simulink model "Demo_DSRC_BSM_Message_cs"  (Simulink 7.6)
settings: Solver=ode5  SolverMode=SingleTasking  StartTime=0.0  StopTime=10  FixedStep=1/20  RelTol=1e-3
model workspace (MAT data in the model file):
  mbox_table.block_array(1).src = 'built-in/Subsystem'
  mbox_table.block_array(1).dest = 'Demo_DSRC_BSM_Message_cs/BMW_Z3_1'
  mbox_table.block_array(1).mode = 0
  mbox_table.block_array(2).src = 'simulink/Sinks/Out1'
  mbox_table.block_array(2).dest = 'Demo_DSRC_BSM_Message_cs/BMW_Z3_1/STATE_BMW_Z3_1'
  mbox_table.block_array(2).mode = 0
  mbox_table.block_array(3).src = 'PreScanSimulinkLibrary/State'
  mbox_table.block_array(3).dest = 'Demo_DSRC_BSM_Message_cs/STATE_BMW_Z3_1'
  mbox_table.block_array(3).mode = 0
  mbox_table.block_array(4).src = 'PreScanSimulinkLibrary/Trajectories'
  mbox_table.block_array(4).dest = 'Demo_DSRC_BSM_Message_cs/BMW_Z3_1/Trajectories'
  mbox_table.block_array(4).mode = 0
  mbox_table.block_array(5).src = 'simulink/Sources/Constant'
  mbox_table.block_array(5).dest = 'Demo_DSRC_BSM_Message_cs/BMW_Z3_1/Trajectories/Trajectory_1_Offset'
  mbox_table.block_array(5).mode = 0
  mbox_table.block_array(6).src = 'PreScanSimulinkLibrary/Trajectory'
  mbox_table.block_array(6).dest = 'Demo_DSRC_BSM_Message_cs/BMW_Z3_1/Trajectories/Trajectory_1'
  mbox_table.block_array(6).mode = 0
  mbox_table.block_array(7).src = 'PreScanSimulinkLibrary/Traj2State'
  mbox_table.block_array(7).dest = 'Demo_DSRC_BSM_Message_cs/BMW_Z3_1/Trajectories/Traj2State1'
  mbox_table.block_array(7).mode = 0
  mbox_table.block_array(8).src = 'simulink/Sinks/Out1'
  mbox_table.block_array(8).dest = 'Demo_DSRC_BSM_Message_cs/BMW_Z3_1/Trajectories/State'
  mbox_table.block_array(8).mode = 0
  mbox_table.block_array(9).src = 'PreScanSimulinkLibrary/SELF'
  mbox_table.block_array(9).dest = 'Demo_DSRC_BSM_Message_cs/SELF_BMW_Z3_1'
  mbox_table.block_array(9).mode = 0
  mbox_table.block_array(10).src = 'simulink/Sources/In1'
  mbox_table.block_array(10).dest = 'Demo_DSRC_BSM_Message_cs/BMW_Z3_1/SELF_BMW_Z3_1'
  mbox_table.block_array(10).mode = 0
  mbox_table.block_array(11).src = 'PreScanSimulinkLibrary/DemuxSELF'
  mbox_table.block_array(11).dest = 'Demo_DSRC_BSM_Message_cs/BMW_Z3_1/SELF_Demux'
  mbox_table.block_array(11).mode = 0
  mbox_table.block_array(12).src = 'PreScanSimulinkLibrary/DSRC_R'
  mbox_table.block_array(12).dest = 'Demo_DSRC_BSM_Message_cs/DSRC_Rx_1'
  mbox_table.block_array(12).mode = 0
  mbox_table.block_array(13).src = 'simulink/Sources/In1'
  mbox_table.block_array(13).dest = 'Demo_DSRC_BSM_Message_cs/BMW_Z3_1/DSRC_Rx_1'
  mbox_table.block_array(13).mode = 0
  mbox_table.block_array(14).src = 'PreScanSimulinkLibrary/DSRC_Receiver'
  mbox_table.block_array(14).dest = 'Demo_DSRC_BSM_Message_cs/BMW_Z3_1/DSRC Receiver'
  mbox_table.block_array(14).mode = 0
  mbox_table.block_array(15).src = 'PreScanSimulinkLibrary/J2735_Decoder_Basic_Safety_Message'
  mbox_table.block_array(15).dest = 'Demo_DSRC_BSM_Message_cs/BMW_Z3_1/J2735 Decoder
    | Basic Safety Message'
  mbox_table.block_array(15).mode = 0
  mbox_table.block_array(16).src = 'built-in/Subsystem'
  mbox_table.block_array(16).dest = 'Demo_DSRC_BSM_Message_cs/Fiat_Bravo_1'
  mbox_table.block_array(16).mode = 0
  mbox_table.block_array(17).src = 'simulink/Sinks/Out1'
  mbox_table.block_array(17).dest = 'Demo_DSRC_BSM_Message_cs/Fiat_Bravo_1/STATE_Fiat_Bravo_1'
  mbox_table.block_array(17).mode = 0
  mbox_table.block_array(18).src = 'PreScanSimulinkLibrary/State'
  mbox_table.block_array(18).dest = 'Demo_DSRC_BSM_Message_cs/STATE_Fiat_Bravo_1'
  mbox_table.block_array(18).mode = 0
  mbox_table.block_array(19).src = 'PreScanSimulinkLibrary/Trajectories'
  mbox_table.block_array(19).dest = 'Demo_DSRC_BSM_Message_cs/Fiat_Bravo_1/Trajectories'
  mbox_table.block_array(19).mode = 0
  mbox_table.block_array(20).src = 'simulink/Sources/Constant'
  mbox_table.block_array(20).dest = 'Demo_DSRC_BSM_Message_cs/Fiat_Bravo_1/Trajectories/Trajectory_2_Offset'
  mbox_table.block_array(20).mode = 0
  mbox_table.block_array(21).src = 'PreScanSimulinkLibrary/Trajectory'
  mbox_table.block_array(21).dest = 'Demo_DSRC_BSM_Message_cs/Fiat_Bravo_1/Trajectories/Trajectory_2'
  mbox_table.block_array(21).mode = 0
  mbox_table.block_array(22).src = 'PreScanSimulinkLibrary/Traj2State'
  mbox_table.block_array(22).dest = 'Demo_DSRC_BSM_Message_cs/Fiat_Bravo_1/Trajectories/Traj2State1'
  mbox_table.block_array(22).mode = 0
  mbox_table.block_array(23).src = 'simulink/Sinks/Out1'
  mbox_table.block_array(23).dest = 'Demo_DSRC_BSM_Message_cs/Fiat_Bravo_1/Trajectories/State'
  mbox_table.block_array(23).mode = 0
  mbox_table.block_array(24).src = 'PreScanSimulinkLibrary/SELF'
  mbox_table.block_array(24).dest = 'Demo_DSRC_BSM_Message_cs/SELF_Fiat_Bravo_1'
  mbox_table.block_array(24).mode = 0
  mbox_table.block_array(25).src = 'simulink/Sources/In1'
  mbox_table.block_array(25).dest = 'Demo_DSRC_BSM_Message_cs/Fiat_Bravo_1/SELF_Fiat_Bravo_1'
  mbox_table.block_array(25).mode = 0
  mbox_table.block_array(26).src = 'PreScanSimulinkLibrary/DemuxSELF'
  mbox_table.block_array(26).dest = 'Demo_DSRC_BSM_Message_cs/Fiat_Bravo_1/SELF_Demux'
  mbox_table.block_array(26).mode = 0
  mbox_table.block_array(27).src = 'PreScanSimulinkLibrary/DSRC_T'
  mbox_table.block_array(27).dest = 'Demo_DSRC_BSM_Message_cs/DSRC_Tx_1'
  mbox_table.block_array(27).mode = 0
  mbox_table.block_array(28).src = 'simulink/Sinks/Out1'
  mbox_table.block_array(28).dest = 'Demo_DSRC_BSM_Message_cs/Fiat_Bravo_1/DSRC_Tx_1'
  mbox_table.block_array(28).mode = 0
  mbox_table.block_array(29).src = 'PreScanSimulinkLibrary/DSRC_Transmitter'
  mbox_table.block_array(29).dest = 'Demo_DSRC_BSM_Message_cs/Fiat_Bravo_1/DSRC Transmitter'
  mbox_table.block_array(29).mode = 0
  mbox_table.block_array(30).src = 'PreScanSimulinkLibrary/J2735_Encoder_Basic_Safety_Message'
  mbox_table.block_array(30).dest = 'Demo_DSRC_BSM_Message_cs/Fiat_Bravo_1/J2735 Encoder
    | Basic Safety Message'
  mbox_table.block_array(30).mode = 0
  mbox_table.block_array(31).src = 'built-in/Subsystem'
  mbox_table.block_array(31).dest = 'Demo_DSRC_BSM_Message_cs/Citroen_C3_1'
  mbox_table.block_array(31).mode = 0
  mbox_table.block_array(32).src = 'simulink/Sinks/Out1'
  mbox_table.block_array(32).dest = 'Demo_DSRC_BSM_Message_cs/Citroen_C3_1/STATE_Citroen_C3_1'
  mbox_table.block_array(32).mode = 0
  mbox_table.block_array(33).src = 'PreScanSimulinkLibrary/State'
  mbox_table.block_array(33).dest = 'Demo_DSRC_BSM_Message_cs/STATE_Citroen_C3_1'
  mbox_table.block_array(33).mode = 0
  mbox_table.block_array(34).src = 'PreScanSimulinkLibrary/Trajectories'
  mbox_table.block_array(34).dest = 'Demo_DSRC_BSM_Message_cs/Citroen_C3_1/Trajectories'
  mbox_table.block_array(34).mode = 0
  mbox_table.block_array(35).src = 'simulink/Sources/Constant'
  mbox_table.block_array(35).dest = 'Demo_DSRC_BSM_Message_cs/Citroen_C3_1/Trajectories/Trajectory_3_Offset'
  mbox_table.block_array(35).mode = 0
  mbox_table.block_array(36).src = 'PreScanSimulinkLibrary/Trajectory'
  mbox_table.block_array(36).dest = 'Demo_DSRC_BSM_Message_cs/Citroen_C3_1/Trajectories/Trajectory_3'
  mbox_table.block_array(36).mode = 0
  mbox_table.block_array(37).src = 'PreScanSimulinkLibrary/Traj2State'
  mbox_table.block_array(37).dest = 'Demo_DSRC_BSM_Message_cs/Citroen_C3_1/Trajectories/Traj2State1'
  mbox_table.block_array(37).mode = 0
  mbox_table.block_array(38).src = 'simulink/Sinks/Out1'
  mbox_table.block_array(38).dest = 'Demo_DSRC_BSM_Message_cs/Citroen_C3_1/Trajectories/State'
  mbox_table.block_array(38).mode = 0
  mbox_table.block_array(39).src = 'PreScanSimulinkLibrary/SELF'
  mbox_table.block_array(39).dest = 'Demo_DSRC_BSM_Message_cs/SELF_Citroen_C3_1'
  mbox_table.block_array(39).mode = 0
  mbox_table.block_array(40).src = 'simulink/Sources/In1'
  mbox_table.block_array(40).dest = 'Demo_DSRC_BSM_Message_cs/Citroen_C3_1/SELF_Citroen_C3_1'
  mbox_table.block_array(40).mode = 0
  mbox_table.block_array(41).src = 'PreScanSimulinkLibrary/DemuxSELF'
  mbox_table.block_array(41).dest = 'Demo_DSRC_BSM_Message_cs/Citroen_C3_1/SELF_Demux'
  mbox_table.block_array(41).mode = 0
  mbox_table.block_array(42).src = 'PreScanSimulinkLibrary/DSRC_T'
  mbox_table.block_array(42).dest = 'Demo_DSRC_BSM_Message_cs/DSRC_Tx_2'
  mbox_table.block_array(42).mode = 0
  mbox_table.block_array(43).src = 'simulink/Sinks/Out1'
  mbox_table.block_array(43).dest = 'Demo_DSRC_BSM_Message_cs/Citroen_C3_1/DSRC_Tx_2'
  mbox_table.block_array(43).mode = 0
  mbox_table.block_array(44).src = 'PreScanSimulinkLibrary/DSRC_Transmitter'
  mbox_table.block_array(44).dest = 'Demo_DSRC_BSM_Message_cs/Citroen_C3_1/DSRC Transmitter'
  mbox_table.block_array(44).mode = 0
  mbox_table.block_array(45).src = 'PreScanSimulinkLibrary/J2735_Encoder_Basic_Safety_Message'
  mbox_table.block_array(45).dest = 'Demo_DSRC_BSM_Message_cs/Citroen_C3_1/J2735 Encoder
    | Basic Safety Message'
  mbox_table.block_array(45).mode = 0
  mbox_table.block_array(46).src = 'SimCoreLibrary/SimCoreConfiguration'
  mbox_table.block_array(46).dest = 'Demo_DSRC_BSM_Message_cs/SimCoreConfiguration'
  mbox_table.block_array(46).mode = 0
  mbox_table.block_array(47).src = 'SimCoreLibrary/Actuators'
  mbox_table.block_array(47).dest = 'Demo_DSRC_BSM_Message_cs/Actuators'
  mbox_table.block_array(47).mode = 0
  mbox_table.block_array(48).src = 'SimCoreLibrary/SetActuators'
  mbox_table.block_array(48).dest = 'Demo_DSRC_BSM_Message_cs/SetActuators'
  mbox_table.block_array(48).mode = 0
  mbox_table.block_array(49).src = 'SimCoreLibrary/GetSensors'
  mbox_table.block_array(49).dest = 'Demo_DSRC_BSM_Message_cs/GetSensors'
  mbox_table.block_array(49).mode = 0
  mbox_table.block_array(50).src = 'SimCoreLibrary/SimCoreInfo'
  mbox_table.block_array(50).dest = 'Demo_DSRC_BSM_Message_cs/SimCoreInfo'
  mbox_table.block_array(50).mode = 0
  mbox_table.block_array(51).src = 'PreScanSimulinkLibrary/Regenerate'
  mbox_table.block_array(51).dest = 'Demo_DSRC_BSM_Message_cs/Regenerate'
  mbox_table.block_array(51).mode = 0
  mbox_table.block_array(52).src = 'PreScanSimulinkLibrary/Record for Replay  '
  mbox_table.block_array(52).dest = 'Demo_DSRC_BSM_Message_cs/Record for Replay  '
  mbox_table.block_array(52).mode = 0
  mbox_table.block_array(53).src = 'PreScanSimulinkLibrary/Open Useful Blocks'
  mbox_table.block_array(53).dest = 'Demo_DSRC_BSM_Message_cs/Open Useful Blocks'
  mbox_table.block_array(53).mode = 0
  mbox_table.block_array(54).src = 'PreScanSimulinkLibrary/PreScan Options   '
  mbox_table.block_array(54).dest = 'Demo_DSRC_BSM_Message_cs/PreScan Options   '
  mbox_table.block_array(54).mode = 0
  mbox_table.block_array(55).src = 'built-in/Note'
  mbox_table.block_array(55).dest = 'Demo_DSRC_BSM_Message_cs/Version:                  '
  mbox_table.block_array(55).mode = 0
  mbox_table.block_array(56).src = 'built-in/Note'
  mbox_table.block_array(56).dest = 'Demo_DSRC_BSM_Message_cs/7.4.0'
  mbox_table.block_array(56).mode = 0
  mbox_table.block_array(57).src = 'built-in/Note'
  mbox_table.block_array(57).dest = 'Demo_DSRC_BSM_Message_cs/Author(s):                '
  mbox_table.block_array(57).mode = 0
  mbox_table.block_array(58).src = 'built-in/Note'
  mbox_table.block_array(58).dest = 'Demo_DSRC_BSM_Message_cs/Jeroen van der Waal'
  mbox_table.block_array(58).mode = 0
  mbox_table.block_array(59).src = 'built-in/Note'
  mbox_table.block_array(59).dest = 'Demo_DSRC_BSM_Message_cs/Descriptive text:      '
  mbox_table.block_array(59).mode = 0
  mbox_table.block_array(60).src = 'built-in/Note'
  mbox_table.block_array(60).dest = 'Demo_DSRC_BSM_Message_cs/Vehicle to Vehicle communication
    | using the DSRC protocol.
    | Only the BSM is supported and it
    | is using the current PreScan
    | Antenna sensor as basis.'
  mbox_table.block_array(60).mode = 0
  mbox_table.block_array(61).src = 'built-in/Note'
  mbox_table.block_array(61).dest = 'Demo_DSRC_BSM_Message_cs/ID
    | 
    | 1
    | 6
    | 7'
  mbox_table.block_array(61).mode = 0
  mbox_table.block_array(62).src = 'built-in/Note'
  mbox_table.block_array(62).dest = 'Demo_DSRC_BSM_Message_cs/OBU-Beacon ID
    | 
    | 
    | 
    | '
  mbox_table.block_array(62).mode = 0
  mbox_table.block_array(63).src = 'built-in/Note'
  mbox_table.block_array(63).dest = 'Demo_DSRC_BSM_Message_cs/TypeID
    | 
    | 1
    | 1
    | 1'
  mbox_table.block_array(63).mode = 0
  mbox_table.block_array(64).src = 'built-in/Note'
  mbox_table.block_array(64).dest = 'Demo_DSRC_BSM_Message_cs/TypeTag
    | 
    | Car
    | Car
    | Car'
  mbox_table.block_array(64).mode = 0
  mbox_table.block_array(65).src = 'built-in/Note'
  mbox_table.block_array(65).dest = 'Demo_DSRC_BSM_Message_cs/SD
    | 
    | Y
    | Y
    | Y'
  mbox_table.block_array(65).mode = 0
  mbox_table.block_array(66).src = 'built-in/Note'
  mbox_table.block_array(66).dest = 'Demo_DSRC_BSM_Message_cs/CD
    | 
    | N
    | N
    | N'
  mbox_table.block_array(66).mode = 0
  mbox_table.block_array(67).src = 'built-in/Note'
  mbox_table.block_array(67).dest = 'Demo_DSRC_BSM_Message_cs/Name
    | 
    | BMW_Z3_1
    | Fiat_Bravo_1
    | Citroen_C3_1'
  mbox_table.block_array(67).mode = 0
  mbox_table.block_array(68).src = 'built-in/Note'
  mbox_table.block_array(68).dest = 'Demo_DSRC_BSM_Message_cs/Num ID       OBU-Beacon ID     Type ID      Type Tag             SD        CD             Name                          '
  mbox_table.block_array(68).mode = 0
  mbox_table.block_index : java.util.Hashtable (value not decoded)
  mbox_table.line_array(1).sys = 'Demo_DSRC_BSM_Message_cs'
  mbox_table.line_array(1).line_id = 'L1'
  mbox_table.line_array(1).iport = 'STATE_BMW_Z3_1/1'
  mbox_table.line_array(1).oport = 'BMW_Z3_1/1'
  mbox_table.line_array(1).mode = 0
  mbox_table.line_array(2).sys = 'Demo_DSRC_BSM_Message_cs/BMW_Z3_1/Trajectories'
  mbox_table.line_array(2).line_id = 'L2'
  mbox_table.line_array(2).iport = 'Traj2State1/1'
  mbox_table.line_array(2).oport = 'Trajectory_1/1'
  mbox_table.line_array(2).mode = 0
  mbox_table.line_array(3).sys = 'Demo_DSRC_BSM_Message_cs/BMW_Z3_1/Trajectories'
  mbox_table.line_array(3).line_id = 'L3'
  mbox_table.line_array(3).iport = 'Traj2State1/2'
  mbox_table.line_array(3).oport = 'Trajectory_1_Offset/1'
  mbox_table.line_array(3).mode = 0
  mbox_table.line_array(4).sys = 'Demo_DSRC_BSM_Message_cs/BMW_Z3_1/Trajectories'
  mbox_table.line_array(4).line_id = 'L4'
  mbox_table.line_array(4).iport = 'State/1'
  mbox_table.line_array(4).oport = 'Traj2State1/1'
  mbox_table.line_array(4).mode = 0
  mbox_table.line_array(5).sys = 'Demo_DSRC_BSM_Message_cs'
  mbox_table.line_array(5).line_id = 'L5'
  mbox_table.line_array(5).iport = 'BMW_Z3_1/1'
  mbox_table.line_array(5).oport = 'SELF_BMW_Z3_1/1'
  mbox_table.line_array(5).mode = 0
  mbox_table.line_array(6).sys = 'Demo_DSRC_BSM_Message_cs/BMW_Z3_1'
  mbox_table.line_array(6).line_id = 'L6'
  mbox_table.line_array(6).iport = 'SELF_Demux/1'
  mbox_table.line_array(6).oport = 'SELF_BMW_Z3_1/1'
  mbox_table.line_array(6).mode = 0
  mbox_table.line_array(7).sys = 'Demo_DSRC_BSM_Message_cs/BMW_Z3_1'
  mbox_table.line_array(7).line_id = 'L7'
  mbox_table.line_array(7).iport = 'J2735 Decoder
    | Basic Safety Message/1'
  mbox_table.line_array(7).oport = 'DSRC Receiver/2'
  mbox_table.line_array(7).mode = 0
  mbox_table.line_array(8).sys = 'Demo_DSRC_BSM_Message_cs/BMW_Z3_1'
  mbox_table.line_array(8).line_id = 'L8'
  mbox_table.line_array(8).iport = 'DSRC Receiver/1'
  mbox_table.line_array(8).oport = 'DSRC_Rx_1/1'
  mbox_table.line_array(8).mode = 0
  mbox_table.line_array(9).sys = 'Demo_DSRC_BSM_Message_cs'
  mbox_table.line_array(9).line_id = 'L9'
  mbox_table.line_array(9).iport = 'BMW_Z3_1/2'
  mbox_table.line_array(9).oport = 'DSRC_Rx_1/1'
  mbox_table.line_array(9).mode = 0
  mbox_table.line_array(10).sys = 'Demo_DSRC_BSM_Message_cs/BMW_Z3_1'
  mbox_table.line_array(10).line_id = 'L10'
  mbox_table.line_array(10).iport = 'STATE_BMW_Z3_1/1'
  mbox_table.line_array(10).oport = 'Trajectories/1'
  mbox_table.line_array(10).mode = 0
  mbox_table.line_array(11).sys = 'Demo_DSRC_BSM_Message_cs'
  mbox_table.line_array(11).line_id = 'L11'
  mbox_table.line_array(11).iport = 'STATE_Fiat_Bravo_1/1'
  mbox_table.line_array(11).oport = 'Fiat_Bravo_1/1'
  mbox_table.line_array(11).mode = 0
  mbox_table.line_array(12).sys = 'Demo_DSRC_BSM_Message_cs/Fiat_Bravo_1/Trajectories'
  mbox_table.line_array(12).line_id = 'L12'
  mbox_table.line_array(12).iport = 'Traj2State1/1'
  mbox_table.line_array(12).oport = 'Trajectory_2/1'
  mbox_table.line_array(12).mode = 0
  mbox_table.line_array(13).sys = 'Demo_DSRC_BSM_Message_cs/Fiat_Bravo_1/Trajectories'
  mbox_table.line_array(13).line_id = 'L13'
  mbox_table.line_array(13).iport = 'Traj2State1/2'
  mbox_table.line_array(13).oport = 'Trajectory_2_Offset/1'
  mbox_table.line_array(13).mode = 0
  mbox_table.line_array(14).sys = 'Demo_DSRC_BSM_Message_cs/Fiat_Bravo_1/Trajectories'
  mbox_table.line_array(14).line_id = 'L14'
  mbox_table.line_array(14).iport = 'State/1'
  mbox_table.line_array(14).oport = 'Traj2State1/1'
  mbox_table.line_array(14).mode = 0
  mbox_table.line_array(15).sys = 'Demo_DSRC_BSM_Message_cs'
  mbox_table.line_array(15).line_id = 'L15'
  mbox_table.line_array(15).iport = 'Fiat_Bravo_1/1'
  mbox_table.line_array(15).oport = 'SELF_Fiat_Bravo_1/1'
  mbox_table.line_array(15).mode = 0
  mbox_table.line_array(16).sys = 'Demo_DSRC_BSM_Message_cs/Fiat_Bravo_1'
  mbox_table.line_array(16).line_id = 'L16'
  mbox_table.line_array(16).iport = 'SELF_Demux/1'
  mbox_table.line_array(16).oport = 'SELF_Fiat_Bravo_1/1'
  mbox_table.line_array(16).mode = 0
  mbox_table.line_array(17).sys = 'Demo_DSRC_BSM_Message_cs/Fiat_Bravo_1'
  mbox_table.line_array(17).line_id = 'L17'
  mbox_table.line_array(17).iport = 'DSRC Transmitter/1'
  mbox_table.line_array(17).oport = 'J2735 Encoder
    | Basic Safety Message/2'
  mbox_table.line_array(17).mode = 0
  mbox_table.line_array(18).sys = 'Demo_DSRC_BSM_Message_cs/Fiat_Bravo_1'
  mbox_table.line_array(18).line_id = 'L18'
  mbox_table.line_array(18).iport = 'DSRC_Tx_1/1'
  mbox_table.line_array(18).oport = 'DSRC Transmitter/1'
  mbox_table.line_array(18).mode = 0
  mbox_table.line_array(19).sys = 'Demo_DSRC_BSM_Message_cs'
  mbox_table.line_array(19).line_id = 'L19'
  mbox_table.line_array(19).iport = 'DSRC_Tx_1/1'
  mbox_table.line_array(19).oport = 'Fiat_Bravo_1/2'
  mbox_table.line_array(19).mode = 0
  mbox_table.line_array(20).sys = 'Demo_DSRC_BSM_Message_cs/Fiat_Bravo_1'
  mbox_table.line_array(20).line_id = 'L20'
  mbox_table.line_array(20).iport = 'STATE_Fiat_Bravo_1/1'
  mbox_table.line_array(20).oport = 'Trajectories/1'
  mbox_table.line_array(20).mode = 0
  mbox_table.line_array(21).sys = 'Demo_DSRC_BSM_Message_cs'
  mbox_table.line_array(21).line_id = 'L21'
  mbox_table.line_array(21).iport = 'STATE_Citroen_C3_1/1'
  mbox_table.line_array(21).oport = 'Citroen_C3_1/1'
  mbox_table.line_array(21).mode = 0
  mbox_table.line_array(22).sys = 'Demo_DSRC_BSM_Message_cs/Citroen_C3_1/Trajectories'
  mbox_table.line_array(22).line_id = 'L22'
  mbox_table.line_array(22).iport = 'Traj2State1/1'
  mbox_table.line_array(22).oport = 'Trajectory_3/1'
  mbox_table.line_array(22).mode = 0
  mbox_table.line_array(23).sys = 'Demo_DSRC_BSM_Message_cs/Citroen_C3_1/Trajectories'
  mbox_table.line_array(23).line_id = 'L23'
  mbox_table.line_array(23).iport = 'Traj2State1/2'
  mbox_table.line_array(23).oport = 'Trajectory_3_Offset/1'
  mbox_table.line_array(23).mode = 0
  mbox_table.line_array(24).sys = 'Demo_DSRC_BSM_Message_cs/Citroen_C3_1/Trajectories'
  mbox_table.line_array(24).line_id = 'L24'
  mbox_table.line_array(24).iport = 'State/1'
  mbox_table.line_array(24).oport = 'Traj2State1/1'
  mbox_table.line_array(24).mode = 0
  mbox_table.line_array(25).sys = 'Demo_DSRC_BSM_Message_cs'
  mbox_table.line_array(25).line_id = 'L25'
  mbox_table.line_array(25).iport = 'Citroen_C3_1/1'
  mbox_table.line_array(25).oport = 'SELF_Citroen_C3_1/1'
  mbox_table.line_array(25).mode = 0
  mbox_table.line_array(26).sys = 'Demo_DSRC_BSM_Message_cs/Citroen_C3_1'
  mbox_table.line_array(26).line_id = 'L26'
  mbox_table.line_array(26).iport = 'SELF_Demux/1'
  mbox_table.line_array(26).oport = 'SELF_Citroen_C3_1/1'
  mbox_table.line_array(26).mode = 0
  mbox_table.line_array(27).sys = 'Demo_DSRC_BSM_Message_cs/Citroen_C3_1'
  mbox_table.line_array(27).line_id = 'L27'
  mbox_table.line_array(27).iport = 'DSRC Transmitter/1'
  mbox_table.line_array(27).oport = 'J2735 Encoder
    | Basic Safety Message/2'
  mbox_table.line_array(27).mode = 0
  mbox_table.line_array(28).sys = 'Demo_DSRC_BSM_Message_cs/Citroen_C3_1'
  mbox_table.line_array(28).line_id = 'L28'
  mbox_table.line_array(28).iport = 'DSRC_Tx_2/1'
  mbox_table.line_array(28).oport = 'DSRC Transmitter/1'
  mbox_table.line_array(28).mode = 0
  mbox_table.line_array(29).sys = 'Demo_DSRC_BSM_Message_cs'
  mbox_table.line_array(29).line_id = 'L29'
  mbox_table.line_array(29).iport = 'DSRC_Tx_2/1'
  mbox_table.line_array(29).oport = 'Citroen_C3_1/2'
  mbox_table.line_array(29).mode = 0
  mbox_table.line_array(30).sys = 'Demo_DSRC_BSM_Message_cs/Citroen_C3_1'
  mbox_table.line_array(30).line_id = 'L30'
  mbox_table.line_array(30).iport = 'STATE_Citroen_C3_1/1'
  mbox_table.line_array(30).oport = 'Trajectories/1'
  mbox_table.line_array(30).mode = 0
  mbox_table.line_index : java.util.Hashtable (value not decoded)
  mbox_table.next_linenr = 31
  mbox_table.next_termlinenr = 1
PreLoadFcn:
  | check_NUTS_defined;
  | 
  | assignin('base',['model_closed_' bdroot],false);
InitFcn:
  | PreScanExperimentInitFcn(bdroot)
StopFcn:
  | PreScanExperimentStopFcn(bdroot)
undefined symbols (not defined in the file): spare_1, spare_10, spare_11, spare_12, spare_13, spare_14, spare_15, spare_16, spare_17, spare_18, spare_19, spare_2, spare_3, spare_4, spare_5, spare_6, spare_7, spare_8, spare_9
libraries: PreScanSimulinkLibrary x12, PreScanUsefulBlocks x4, simulink x2
(part 1 of 3)
CloseFcn:
  | evalin('base',['clear model_closed_' bdroot]);
settings Model: Creator=PRESCAN  LastModifiedBy=buildbot
settings OptimizationCC: InitFltsAndDblsToZero=on
settings DebuggingCC: SaveWithParameterizedLinksMsg=none  SignalResolutionControl=TryResolveAllWithWarning  SolverPrmCheckMsg=none  MultiTaskDSMMsg=warning  MultiTaskCondExecSysMsg=none  SimStateInterfaceChecksumMismatchMsg=none
settings SFSimCC: SimParseCustomCode=off
settings RTWCC: IncludeERTFirstTime=on
settings GRTTargetCC: TargetFcnLib=ansi_tfl_tmw.mat

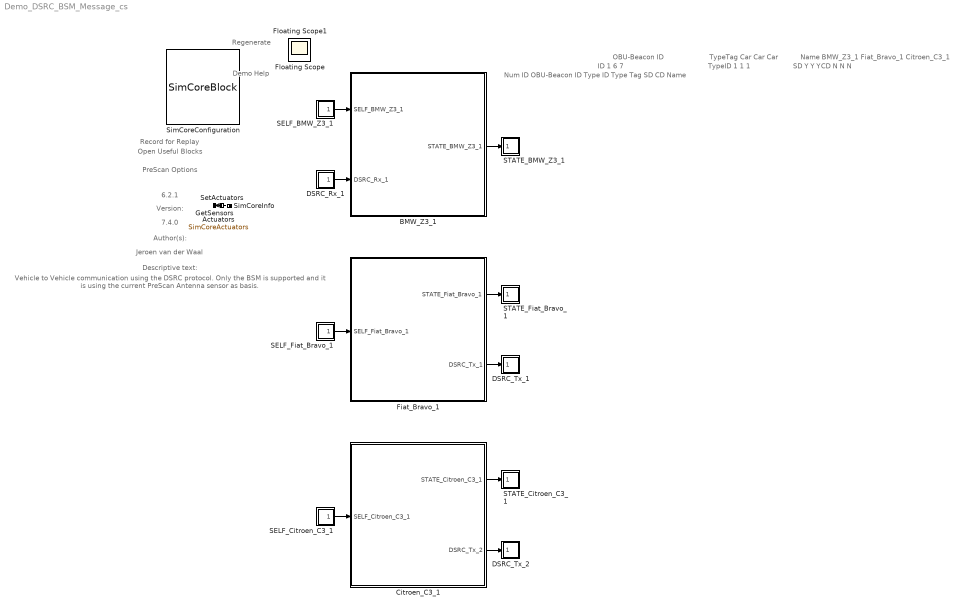
== system Demo_DSRC_BSM_Message_cs ==
  note: 6.2.1
  note: Demo Help
  note: Regenerate
  note: Record for Replay
  note: Open Useful Blocks
  note: PreScan Options
  note: Version:
  note: 7.4.0
  note: Author(s):
  note: Jeroen van der Waal
  note: Descriptive text:
  note: Vehicle to Vehicle communication
      | using the DSRC protocol.
      | Only the BSM is supported and it
      | is using the current PreScan
      | Antenna sensor as basis.
  note: ID
      |
      | 1
      | 6
      | 7
  note: OBU-Beacon ID
  note: TypeID
      |
      | 1
      | 1
      | 1
  note: TypeTag
      |
      | Car
      | Car
      | Car
  note: SD
      |
      | Y
      | Y
      | Y
  note: CD
      |
      | N
      | N
      | N
  note: Name
      |
      | BMW_Z3_1
      | Fiat_Bravo_1
      | Citroen_C3_1
  note: Num ID OBU-Beacon ID Type ID Type Tag SD CD Name
  Actuators : DataStoreMemory  Tag=Actuators  DataStoreName=SimCoreActuators  InitialValue=zeros(93,1)
      settings: DeleteFcn=PreScanBlockDeleteFcn;
  BMW_Z3_1 : Subsystem  Tag=WorldObjectSubSystem  InitFcn=UniqueId = '16';
      mask Display: image(imread('BMW_Z3.jpg'));color('white');text(0,0,' ID=1\n')
  Citroen_C3_1 : Subsystem  Tag=WorldObjectSubSystem  InitFcn=UniqueId = '29';
      mask Display: image(imread('Citroen_C3.jpg'));color('white');text(0,0,' ID=7\n')
  DSRC_Rx_1 : Subsystem  Tag=DSRC_R  Priority=3  mask(PreScan Source Block: DSRC Receiver){NrEntitiesOut=2, PortName=DSRC_Rx_1, PortIndex=8, PortWidth=94, TimeStep=1/20}
      mask prompts: NrEntitiesOut "User Specified: # of Visible Actors"; PortName "Auto Assigned: Port Name [-]"; PortIndex "Auto Assigned: Index [-]"; PortWidth "Auto Assigned: Port Dimensions [-]"; TimeStep "Auto Assigned: Upload Period [s]"
      mask help:
      | Using the DSRC Receiver (R) and Transmitter (T) information between actors can be exchanged.
      |
      | The DSRC Reciever receives actor information.
      |
      | For more information, please click Help.
      settings: DeleteFcn=PreScanBlockDeleteFcn;
      mask Help: eval('openHelp(473)')
      mask Display: image(imread('DSRCReceiver.png'))
  DSRC_Tx_1 : Subsystem  Tag=DSRC_T  Priority=0  mask(PreScan Sink Block: DSRC_T){PortName=DSRC_Tx_1, PortIndex=30, PortWidth=24, TimeStep=1/20}
      mask prompts: PortName "Auto Assigned: Port Name [-]"; PortIndex "Auto Assigned: Index [-]"; PortWidth "Auto Assigned: Port Dimensions [-]"; TimeStep "Auto Assigned: Upload Period [s]"
      mask help:
      | Using the DSRC Receiver and Transmitter information between actors can be exchanged.
      |
      | The DSRC Transmitter receives actors information.
      |
      | For more information, please click Help.
      settings: DeleteFcn=PreScanBlockDeleteFcn;
      mask Help: eval('openHelp(473)')
      mask Display: image(imread('DSRCTransmitter.png'))
  DSRC_Tx_2 : Subsystem  Tag=DSRC_T  Priority=0  mask(PreScan Sink Block: DSRC_T){PortName=DSRC_Tx_2, PortIndex=69, PortWidth=24, TimeStep=1/20}
      mask prompts: PortName "Auto Assigned: Port Name [-]"; PortIndex "Auto Assigned: Index [-]"; PortWidth "Auto Assigned: Port Dimensions [-]"; TimeStep "Auto Assigned: Upload Period [s]"
      mask help:
      | Using the DSRC Receiver and Transmitter information between actors can be exchanged.
      |
      | The DSRC Transmitter receives actors information.
      |
      | For more information, please click Help.
      settings: DeleteFcn=PreScanBlockDeleteFcn;
      mask Help: eval('openHelp(473)')
      mask Display: image(imread('DSRCTransmitter.png'))
  Fiat_Bravo_1 : Subsystem  Tag=WorldObjectSubSystem  InitFcn=UniqueId = '21';
      mask Display: image(imread('Fiat_Bravo.jpg'));color('white');text(0,0,' ID=6\n')
  GetSensors : Subsystem  Tag=GetSensors  Priority=2  mask(PreScan Simulation Core Block){NrOfSensors=118, TimeStep=1/20}
      mask prompts: NrOfSensors "Number of sensor values"; TimeStep "Timestep [s]"
      mask help:
      | Please do not remove this block from the PreScan compilation sheet,
      | as it contains essential configuration parameters for a PreScan simulation.
      settings: DeleteFcn=PreScanBlockDeleteFcn;
  SELF_BMW_Z3_1 : Subsystem  Tag=SELF  Priority=3  mask(PreScan Source Block: SELF){PortName=SELF_BMW_Z3_1, PortIndex=0, PortWidth=8, TimeStep=1/20}
      mask prompts: PortName "Auto-Assigned: Port Name [-]"; PortIndex "Auto-Assigned: Port Index [-]"; PortWidth "Auto-Assigned: Port Dimensions"; TimeStep "Auto-Assigned: Upload Period [s]"
      mask help:
      | The SELF port shows (state) information of the actor itself. The outputs are position in the experiment's axis system and the GPS coordinates, and the object's absolute velocity and compass heading.
      |
      | For more information, please click Help.
      settings: DeleteFcn=PreScanBlockDeleteFcn;
      mask Help: eval('openHelp(462)')
      mask Display: image(imread('GPS.png'))
  SELF_Citroen_C3_1 : Subsystem  Tag=SELF  Priority=3  mask(PreScan Source Block: SELF){PortName=SELF_Citroen_C3_1, PortIndex=110, PortWidth=8, TimeStep=1/20}
      mask prompts: PortName "Auto-Assigned: Port Name [-]"; PortIndex "Auto-Assigned: Port Index [-]"; PortWidth "Auto-Assigned: Port Dimensions"; TimeStep "Auto-Assigned: Upload Period [s]"
      mask help:
      | The SELF port shows (state) information of the actor itself. The outputs are position in the experiment's axis system and the GPS coordinates, and the object's absolute velocity and compass heading.
      |
      | For more information, please click Help.
      settings: DeleteFcn=PreScanBlockDeleteFcn;
      mask Help: eval('openHelp(462)')
      mask Display: image(imread('GPS.png'))
  SELF_Fiat_Bravo_1 : Subsystem  Tag=SELF  Priority=3  mask(PreScan Source Block: SELF){PortName=SELF_Fiat_Bravo_1, PortIndex=102, PortWidth=8, TimeStep=1/20}
      mask prompts: PortName "Auto-Assigned: Port Name [-]"; PortIndex "Auto-Assigned: Port Index [-]"; PortWidth "Auto-Assigned: Port Dimensions"; TimeStep "Auto-Assigned: Upload Period [s]"
      mask help:
      | The SELF port shows (state) information of the actor itself. The outputs are position in the experiment's axis system and the GPS coordinates, and the object's absolute velocity and compass heading.
      |
      | For more information, please click Help.
      settings: DeleteFcn=PreScanBlockDeleteFcn;
      mask Help: eval('openHelp(462)')
      mask Display: image(imread('GPS.png'))
  STATE_BMW_Z3_1 : Subsystem  Tag=State  Priority=0  mask(PreScan Sink Block: State){x0=1.5151519775390623, y0=56.40850830078125, z0=0.4784, Roll0=0, Pitch0=0, Yaw0=0, TimeStep=1/20}
      mask prompts: x0 "Ini x-position VEHICLE wrt GLOBAL axis system [m]"; y0 "Ini y-position VEHICLE wrt GLOBAL axis system [m]"; z0 "Ini z-position VEHICLE wrt GLOBAL axis system [m]"; Roll0 "Ini roll-angle BODY wrt VEHICLE axis system [deg]"; Pitch0 "Ini pitch-angle BODY wrt VEHICLE axis system [deg]"; Yaw0 "Ini yaw-angle VEHICLE wrt GLOBAL axis system [deg]"; TimeStep "Time Step [s]"
      mask help:
      | The Actor State contains a vector signal of size (9x1), containing the following signals:
      |
      | -  Position                  (x,y,z)                                     [m]
      | -  Velocity                  (vx,vy,vz)                               [m/s]
      | -  Angles                    (Roll, Pitch, Yaw)                   [rad]
      |
      | The Actor state is defined in the global axis system.
      | The state is superponed on the Initial position defined in the GUI.
      |
      | For more information, please click Help.
      settings: DeleteFcn=PreScanBlockDeleteFcn;
      mask Help: eval('openHelp(222)')
      mask Display: image(imread('State.png'))
  STATE_Citroen_C3_1 : Subsystem  Tag=State  Priority=0  mask(PreScan Sink Block: State){x0=81.265151977539063, y0=20.15850830078125, z0=0.58, Roll0=0, Pitch0=0, Yaw0=90, TimeStep=1/20}
      mask prompts: x0 "Ini x-position VEHICLE wrt GLOBAL axis system [m]"; y0 "Ini y-position VEHICLE wrt GLOBAL axis system [m]"; z0 "Ini z-position VEHICLE wrt GLOBAL axis system [m]"; Roll0 "Ini roll-angle BODY wrt VEHICLE axis system [deg]"; Pitch0 "Ini pitch-angle BODY wrt VEHICLE axis system [deg]"; Yaw0 "Ini yaw-angle VEHICLE wrt GLOBAL axis system [deg]"; TimeStep "Time Step [s]"
      mask help:
      | The Actor State contains a vector signal of size (9x1), containing the following signals:
      |
      | -  Position                  (x,y,z)                                     [m]
      | -  Velocity                  (vx,vy,vz)                               [m/s]
      | -  Angles                    (Roll, Pitch, Yaw)                   [rad]
      |
      | The Actor state is defined in the global axis system.
      | The state is superponed on the Initial position defined in the GUI.
      |
      | For more information, please click Help.
      settings: DeleteFcn=PreScanBlockDeleteFcn;
      mask Help: eval('openHelp(222)')
      mask Display: image(imread('State.png'))
  STATE_Fiat_Bravo_1 : Subsystem  Tag=State  Priority=0  mask(PreScan Sink Block: State){x0=81.265151977539063, y0=10.15850830078125, z0=0.55, Roll0=0, Pitch0=0, Yaw0=90, TimeStep=1/20}
      mask prompts: x0 "Ini x-position VEHICLE wrt GLOBAL axis system [m]"; y0 "Ini y-position VEHICLE wrt GLOBAL axis system [m]"; z0 "Ini z-position VEHICLE wrt GLOBAL axis system [m]"; Roll0 "Ini roll-angle BODY wrt VEHICLE axis system [deg]"; Pitch0 "Ini pitch-angle BODY wrt VEHICLE axis system [deg]"; Yaw0 "Ini yaw-angle VEHICLE wrt GLOBAL axis system [deg]"; TimeStep "Time Step [s]"
      mask help:
      | The Actor State contains a vector signal of size (9x1), containing the following signals:
      |
      | -  Position                  (x,y,z)                                     [m]
      | -  Velocity                  (vx,vy,vz)                               [m/s]
      | -  Angles                    (Roll, Pitch, Yaw)                   [rad]
      |
      | The Actor state is defined in the global axis system.
      | The state is superponed on the Initial position defined in the GUI.
      |
      | For more information, please click Help.
      settings: DeleteFcn=PreScanBlockDeleteFcn;
      mask Help: eval('openHelp(222)')
      mask Display: image(imread('State.png'))
  SetActuators : Subsystem  Tag=SetActuators  Priority=1  mask(PreScan Simulation Core Block){TimeStep=1/20, NrOfActuators=93}
      mask prompts: TimeStep "Timestep [s]"; NrOfActuators "Number of actuator values"
      mask help:
      | Please do not remove this block from the PreScan compilation sheet,
      | as it contains essential configuration parameters for a PreScan simulation.
      settings: DeleteFcn=PreScanBlockDeleteFcn;
  SimCoreConfiguration : M-S-Function  Tag=SimCoreConfiguration  Description=42FCA56BF979A3B97F74E9F89DAF0EF71980342D3A192C78BBA9A4C6F392A223  FunctionName=SimCoreBlock  Parameters=ExperimentXML PortsXML SimulationCore HostName CheckStart EnableLog RfR EnableGPUAccel ShowComputationTime  mask(PreScan Simulation Core Configurator){SimulationCore=NUTS, HostName=0, CheckStart=0, prescanversion='7.4.0', EnableLog=off, RfR=0, EnableGPUAccel=off, ShowComputationTime=off}
      mask prompts: SimulationCore "Simulation Core"; HostName "Simulation Host"; CheckStart "Show START Dialog"; prescanversion "PreScan Version"; EnableLog "Create TA Log"; RfR "Record for Replay"; EnableGPUAccel "Enable GPU Acceleration"; ShowComputationTime "Show ComputationTime Scope"
      mask help:
      | Please do not remove this block from the PreScan compilation sheet,
      | as it contains essential configuration parameter for a PreScan simulation.
      mask init:
      | model = bdroot;
      | ExperimentXML = [model(1:end-3) '.pex'];
      | PortsXML = [model '_ports.pcd'];
      settings: DeleteFcn=PreScanBlockDeleteFcn;  ModelCloseFcn=assignin('base',['model_closed_' bdroot],true);
      mask Help: eval('openHelp(812)')
      mask Display: image(imread('prescanlogo.ico'))
  SimCoreInfo : Subsystem  Tag=SimCoreInfo
  Floating Scope : Scope
      settings: Floating=on
  Floating Scope1 : Scope
      settings: Floating=on  SaveName=ScopeData2
  wires:
  BMW_Z3_1/1(STATE_BMW_Z3_1) -> STATE_BMW_Z3_1/1(State)
  SELF_BMW_Z3_1/1(U) -> BMW_Z3_1/1(SELF_BMW_Z3_1)
  DSRC_Rx_1/1(U) -> BMW_Z3_1/2(DSRC_Rx_1)
  Fiat_Bravo_1/1(STATE_Fiat_Bravo_1) -> STATE_Fiat_Bravo_1/1(State)
  SELF_Fiat_Bravo_1/1(U) -> Fiat_Bravo_1/1(SELF_Fiat_Bravo_1)
  Fiat_Bravo_1/2(DSRC_Tx_1) -> DSRC_Tx_1/1(Y)
  Citroen_C3_1/1(STATE_Citroen_C3_1) -> STATE_Citroen_C3_1/1(State)
  SELF_Citroen_C3_1/1(U) -> Citroen_C3_1/1(SELF_Citroen_C3_1)
  Citroen_C3_1/2(DSRC_Tx_2) -> DSRC_Tx_2/1(Y)
  SetActuators/1(dummy) -> GetSensors/1(dummy)

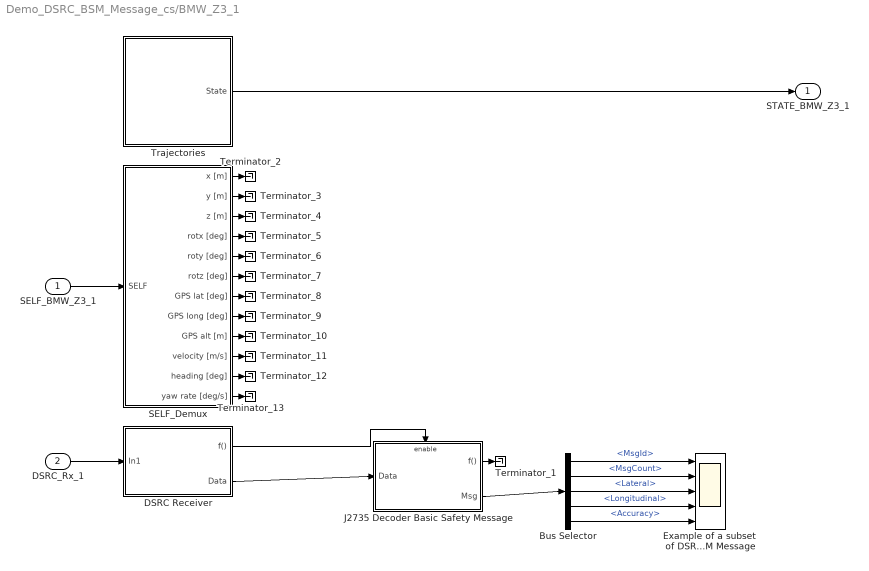
== system Demo_DSRC_BSM_Message_cs/BMW_Z3_1 ==
  SELF_BMW_Z3_1 : Inport  Tag=SELFInport
  DSRC_Rx_1 : Inport  Tag=DSRC_RInport  Port=2
  Bus Selector : BusSelector  OutputSignals=MsgId,MsgCount,Lateral,Longitudinal,Accuracy
  DSRC Receiver : Subsystem  Tag=DSRC_Receiver
  Example of a subset  of DSRC Receiver BSM Message : Scope  NumInputPorts=5
      settings: TimeRange=10  YMin=0~0~0~0~0  YMax=2~150~6000~8000~80000  MaxDataPoints=50000
  J2735 Decoder Basic Safety Message : Subsystem  Tag=J2735_Decoder_Basic_Safety_Message
  SELF_Demux : Subsystem  Tag=DemuxSELF
      settings: DeleteFcn=PreScanBlockDeleteFcn;
      mask Type: PreScan Demux Block:
      mask Display:
      | port_label('output',1,'x [m]')
      | port_label('output',2,'y [m]')
      | port_label('output',3,'z [m]','texmode','on')
      | port_label('output',4,'Rotx [deg]','texmode','on')
      | port_label('output',5,'Roty [deg]','texmode','on')
      | port_label('output',6,'Rotz [deg]','texmode','on')
      | port_label('output',7,'GPS lat [deg]','texmode','on')
      | port_label('output',8,'GPS long [deg]','texmode','on')
      | port_label('output',9,'GPS alt [m]','texmode','on')
      | port_label('output',10,'Velocity [m/s]')
      | port_label('output',11,'Heading [deg]')
      | port_label('output',12,'Yaw rate [deg/s]')
  Terminator_{1..13} (13 alike) : Terminator
  Trajectories : Subsystem  Tag=Trajectories
      settings: DeleteFcn=PreScanBlockDeleteFcn;
      mask Type: PreScan Source Block: Trajectories
      mask Description:
      | The Trajectory block contains the trajectories defined in the PreScan Experiment Editor. The output of the trajectory block is the (vehicle) State.
      | 
      | For more information, please click Help.
      mask Help: eval('openHelp(312)')
      mask Display: image(imread('Trajectory.png'));
  STATE_BMW_Z3_1 : Outport  Tag=StateOutport
  wires:
  Bus Selector/1 -> Example of a subset  of DSRC Receiver BSM Message/1  "<MsgId>"
  Bus Selector/2 -> Example of a subset  of DSRC Receiver BSM Message/2  "<MsgCount>"
  Bus Selector/3 -> Example of a subset  of DSRC Receiver BSM Message/3  "<Lateral>"
  Bus Selector/4 -> Example of a subset  of DSRC Receiver BSM Message/4  "<Longitudinal>"
  Bus Selector/5 -> Example of a subset  of DSRC Receiver BSM Message/5  "<Accuracy>"
  SELF_BMW_Z3_1/1 -> SELF_Demux/1(SELF)
  DSRC Receiver/1(f()) -> J2735 Decoder Basic Safety Message/Enable
  DSRC Receiver/2(Data) -> J2735 Decoder Basic Safety Message/1(Data)
  DSRC_Rx_1/1 -> DSRC Receiver/1(In1)
  Trajectories/1(State) -> STATE_BMW_Z3_1/1
  J2735 Decoder Basic Safety Message/2(Msg) -> Bus Selector/1
  J2735 Decoder Basic Safety Message/1(f()) -> Terminator_1/1
  SELF_Demux/1(x [m]) -> Terminator_2/1
  SELF_Demux/2(y [m]) -> Terminator_3/1
  SELF_Demux/3(z [m]) -> Terminator_4/1
  SELF_Demux/4(rotx [deg]) -> Terminator_5/1
  SELF_Demux/5(roty [deg]) -> Terminator_6/1
  SELF_Demux/6(rotz [deg]) -> Terminator_7/1
  SELF_Demux/7(GPS lat [deg]) -> Terminator_8/1
  SELF_Demux/8(GPS long [deg]) -> Terminator_9/1
  SELF_Demux/9(GPS alt [m]) -> Terminator_10/1
  SELF_Demux/10(velocity [m/s]) -> Terminator_11/1
  SELF_Demux/11(heading [deg]) -> Terminator_12/1
  SELF_Demux/12(yaw rate [deg/s]) -> Terminator_13/1

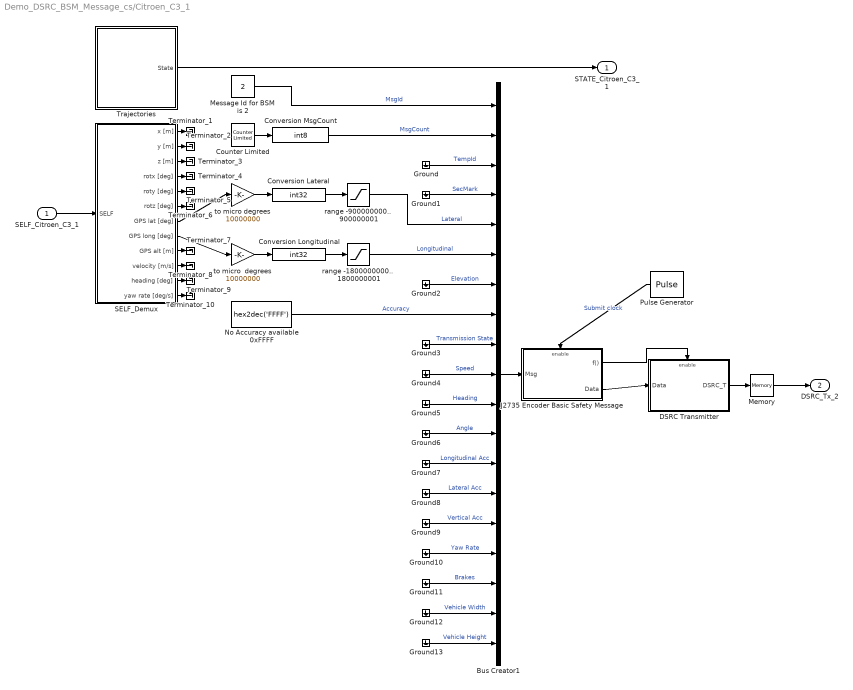
== system Demo_DSRC_BSM_Message_cs/Citroen_C3_1 ==
  SELF_Citroen_C3_1 : Inport  Tag=SELFInport
  Bus Creator1 : BusCreator  Inputs=19
  Conversion Lateral : DataTypeConversion  OutDataTypeStr=int32
  Conversion Longitudinal : DataTypeConversion  OutDataTypeStr=int32
  Conversion MsgCount : DataTypeConversion  OutDataTypeStr=int8
  Counter Limited : simulink/Sources/Counter Limited  SystemSampleTime=-1  uplimit=127  tsamp=-1
  DSRC Transmitter : Subsystem  Tag=DSRC_Transmitter
  Ground{,1..13} (14 alike) : Ground
  J2735 Encoder Basic Safety Message : Subsystem  Tag=J2735_Encoder_Basic_Safety_Message
  Memory : Memory
  Message Id for BSM is 2 : Constant  Value=2  OutDataTypeStr=int8
  No Accuracy available 0xFFFF : Constant  Value=hex2dec('FFFF')  OutDataTypeStr=int32
  Pulse Generator : DiscretePulseGenerator  Period=1  SampleTime=1/20
  SELF_Demux : Subsystem  Tag=DemuxSELF
      settings: DeleteFcn=PreScanBlockDeleteFcn;
      mask Type: PreScan Demux Block:
      mask Display:
      | port_label('output',1,'x [m]')
      | port_label('output',2,'y [m]')
      | port_label('output',3,'z [m]','texmode','on')
      | port_label('output',4,'Rotx [deg]','texmode','on')
      | port_label('output',5,'Roty [deg]','texmode','on')
      | port_label('output',6,'Rotz [deg]','texmode','on')
      | port_label('output',7,'GPS lat [deg]','texmode','on')
      | port_label('output',8,'GPS long [deg]','texmode','on')
      | port_label('output',9,'GPS alt [m]','texmode','on')
      | port_label('output',10,'Velocity [m/s]')
      | port_label('output',11,'Heading [deg]')
      | port_label('output',12,'Yaw rate [deg/s]')
  Terminator_{1..10} (10 alike) : Terminator
  Trajectories : Subsystem  Tag=Trajectories
      settings: DeleteFcn=PreScanBlockDeleteFcn;
      mask Type: PreScan Source Block: Trajectories
      mask Description:
      | The Trajectory block contains the trajectories defined in the PreScan Experiment Editor. The output of the trajectory block is the (vehicle) State.
      | 
      | For more information, please click Help.
      mask Help: eval('openHelp(312)')
      mask Display: image(imread('Trajectory.png'));
  range -1800000000..  1800000001 : Saturate  UpperLimit=1800000001  LowerLimit=-1800000000  OutDataTypeStr=int32
  range -900000000..  900000001 : Saturate  UpperLimit=900000001  LowerLimit=-900000000  OutDataTypeStr=int32
  to micro degrees : Gain  Gain=10000000
  to micro  degrees : Gain  Gain=10000000
  STATE_Citroen_C3_1 : Outport  Tag=StateOutport
  DSRC_Tx_2 : Outport  Tag=DSRC_TOutport  Port=2
  wires:
  Message Id for BSM is 2/1 -> Bus Creator1/1  "MsgId"
  Counter Limited/1 -> Conversion MsgCount/1
  to micro  degrees/1 -> Conversion Longitudinal/1
  Conversion Longitudinal/1 -> range -1800000000..  1800000001/1
  Conversion Lateral/1 -> range -900000000..  900000001/1
  to micro degrees/1 -> Conversion Lateral/1
  No Accuracy available 0xFFFF/1 -> Bus Creator1/8  "Accuracy"
  Ground13/1 -> Bus Creator1/19  "Vehicle Height"
  Ground12/1 -> Bus Creator1/18  "Vehicle Width"
  Ground11/1 -> Bus Creator1/17  "Brakes"
  Ground10/1 -> Bus Creator1/16  "Yaw Rate"
  Ground9/1 -> Bus Creator1/15  "Vertical Acc"
  Ground8/1 -> Bus Creator1/14  "Lateral Acc"
  Ground7/1 -> Bus Creator1/13  "Longitudinal Acc"
  Ground6/1 -> Bus Creator1/12  "Angle"
  Ground5/1 -> Bus Creator1/11  "Heading"
  Ground4/1 -> Bus Creator1/10  "Speed"
  Ground3/1 -> Bus Creator1/9  "Transmission State"
  Ground2/1 -> Bus Creator1/7  "Elevation"
  Ground1/1 -> Bus Creator1/4  "SecMark"
  Ground/1 -> Bus Creator1/3  "TempId"
  Conversion MsgCount/1 -> Bus Creator1/2  "MsgCount"
  range -900000000..  900000001/1 -> Bus Creator1/5  "Lateral"
  range -1800000000..  1800000001/1 -> Bus Creator1/6  "Longitudinal"
  SELF_Citroen_C3_1/1 -> SELF_Demux/1(SELF)
  J2735 Encoder Basic Safety Message/1(f()) -> DSRC Transmitter/Enable
  J2735 Encoder Basic Safety Message/2(Data) -> DSRC Transmitter/1(Data)
  DSRC Transmitter/1(DSRC_T) -> Memory/1
  Trajectories/1(State) -> STATE_Citroen_C3_1/1
  SELF_Demux/8(GPS long [deg]) -> to micro  degrees/1
  Bus Creator1/1 -> J2735 Encoder Basic Safety Message/1(Msg)
  SELF_Demux/7(GPS lat [deg]) -> to micro degrees/1
  SELF_Demux/1(x [m]) -> Terminator_1/1
  SELF_Demux/2(y [m]) -> Terminator_2/1
  SELF_Demux/3(z [m]) -> Terminator_3/1
  SELF_Demux/4(rotx [deg]) -> Terminator_4/1
  SELF_Demux/5(roty [deg]) -> Terminator_5/1
  SELF_Demux/6(rotz [deg]) -> Terminator_6/1
  SELF_Demux/9(GPS alt [m]) -> Terminator_7/1
  SELF_Demux/10(velocity [m/s]) -> Terminator_8/1
  SELF_Demux/11(heading [deg]) -> Terminator_9/1
  SELF_Demux/12(yaw rate [deg/s]) -> Terminator_10/1
  Pulse Generator/1 -> J2735 Encoder Basic Safety Message/Enable  "Submit clock"
  Memory/1 -> DSRC_Tx_2/1

== system Demo_DSRC_BSM_Message_cs/DSRC_Rx_1 ==
  Selector : Selector  IndexMode=Zero-based  IndexOptions=Starting index (dialog)  Indices=PortIndex  OutputSizes=PortWidth(1)
  U : Outport
  wires:
  [SimCoreSensors] -> Selector/1
  Selector/1 -> U/1

== system Demo_DSRC_BSM_Message_cs/DSRC_Tx_1 ==
  Y : Inport  SampleTime=TimeStep
  Assignment : Assignment  IndexMode=Zero-based  SampleTime=TimeStep  IndexOptions=Starting index (dialog)  Indices=PortIndex  OutputSizes=[1 1]
  Data Store Read : DataStoreRead  DataStoreName=SimCoreActuators  SampleTime=TimeStep
  Data Store Write : DataStoreWrite  DataStoreName=SimCoreActuators
  wires:
  Y/1 -> Assignment/2
  Data Store Read/1 -> Assignment/1
  Assignment/1 -> Data Store Write/1

== system Demo_DSRC_BSM_Message_cs/DSRC_Tx_2 ==
  Y : Inport  SampleTime=TimeStep
  Assignment : Assignment  IndexMode=Zero-based  SampleTime=TimeStep  IndexOptions=Starting index (dialog)  Indices=PortIndex  OutputSizes=[1 1]
  Data Store Read : DataStoreRead  DataStoreName=SimCoreActuators  SampleTime=TimeStep
  Data Store Write : DataStoreWrite  DataStoreName=SimCoreActuators
  wires:
  Y/1 -> Assignment/2
  Data Store Read/1 -> Assignment/1
  Assignment/1 -> Data Store Write/1

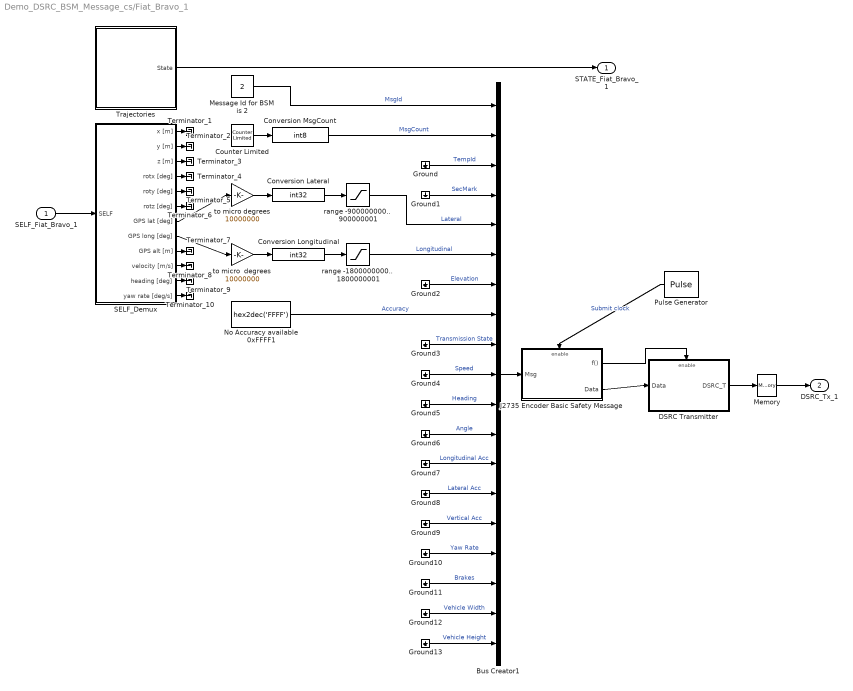
== system Demo_DSRC_BSM_Message_cs/Fiat_Bravo_1 ==
  SELF_Fiat_Bravo_1 : Inport  Tag=SELFInport
  Bus Creator1 : BusCreator  Inputs=19
  Conversion Lateral : DataTypeConversion  OutDataTypeStr=int32
  Conversion Longitudinal : DataTypeConversion  OutDataTypeStr=int32
  Conversion MsgCount : DataTypeConversion  OutDataTypeStr=int8
  Counter Limited : simulink/Sources/Counter Limited  SystemSampleTime=-1  uplimit=127  tsamp=-1
  DSRC Transmitter : Subsystem  Tag=DSRC_Transmitter
  Ground{,1..13} (14 alike) : Ground
  J2735 Encoder Basic Safety Message : Subsystem  Tag=J2735_Encoder_Basic_Safety_Message
  Memory : Memory
  Message Id for BSM is 2 : Constant  Value=2  OutDataTypeStr=int8
  No Accuracy available 0xFFFF1 : Constant  Value=hex2dec('FFFF')  OutDataTypeStr=int32
  Pulse Generator : DiscretePulseGenerator  Period=1  SampleTime=1/20
  SELF_Demux : Subsystem  Tag=DemuxSELF
      settings: DeleteFcn=PreScanBlockDeleteFcn;
      mask Type: PreScan Demux Block:
      mask Display:
      | port_label('output',1,'x [m]')
      | port_label('output',2,'y [m]')
      | port_label('output',3,'z [m]','texmode','on')
      | port_label('output',4,'Rotx [deg]','texmode','on')
      | port_label('output',5,'Roty [deg]','texmode','on')
      | port_label('output',6,'Rotz [deg]','texmode','on')
      | port_label('output',7,'GPS lat [deg]','texmode','on')
      | port_label('output',8,'GPS long [deg]','texmode','on')
      | port_label('output',9,'GPS alt [m]','texmode','on')
      | port_label('output',10,'Velocity [m/s]')
      | port_label('output',11,'Heading [deg]')
      | port_label('output',12,'Yaw rate [deg/s]')
  Terminator_{1..10} (10 alike) : Terminator
  Trajectories : Subsystem  Tag=Trajectories
      settings: DeleteFcn=PreScanBlockDeleteFcn;
      mask Type: PreScan Source Block: Trajectories
      mask Description:
      | The Trajectory block contains the trajectories defined in the PreScan Experiment Editor. The output of the trajectory block is the (vehicle) State.
      | 
      | For more information, please click Help.
      mask Help: eval('openHelp(312)')
      mask Display: image(imread('Trajectory.png'));
  range -1800000000..  1800000001 : Saturate  UpperLimit=1800000001  LowerLimit=-1800000000  OutDataTypeStr=int32
  range -900000000..  900000001 : Saturate  UpperLimit=900000001  LowerLimit=-900000000  OutDataTypeStr=int32
  to micro degrees : Gain  Gain=10000000
  to micro  degrees : Gain  Gain=10000000
  STATE_Fiat_Bravo_1 : Outport  Tag=StateOutport
  DSRC_Tx_1 : Outport  Tag=DSRC_TOutport  Port=2
  wires:
  Message Id for BSM is 2/1 -> Bus Creator1/1  "MsgId"
  Counter Limited/1 -> Conversion MsgCount/1
  to micro  degrees/1 -> Conversion Longitudinal/1
  Conversion Longitudinal/1 -> range -1800000000..  1800000001/1
  Conversion Lateral/1 -> range -900000000..  900000001/1
  to micro degrees/1 -> Conversion Lateral/1
  No Accuracy available 0xFFFF1/1 -> Bus Creator1/8  "Accuracy"
  Ground13/1 -> Bus Creator1/19  "Vehicle Height"
  Ground12/1 -> Bus Creator1/18  "Vehicle Width"
  Ground11/1 -> Bus Creator1/17  "Brakes"
  Ground10/1 -> Bus Creator1/16  "Yaw Rate"
  Ground9/1 -> Bus Creator1/15  "Vertical Acc"
  Ground8/1 -> Bus Creator1/14  "Lateral Acc"
  Ground7/1 -> Bus Creator1/13  "Longitudinal Acc"
  Ground6/1 -> Bus Creator1/12  "Angle"
  Ground5/1 -> Bus Creator1/11  "Heading"
  Ground4/1 -> Bus Creator1/10  "Speed"
  Ground3/1 -> Bus Creator1/9  "Transmission State"
  Ground2/1 -> Bus Creator1/7  "Elevation"
  Ground1/1 -> Bus Creator1/4  "SecMark"
  Ground/1 -> Bus Creator1/3  "TempId"
  Conversion MsgCount/1 -> Bus Creator1/2  "MsgCount"
  range -900000000..  900000001/1 -> Bus Creator1/5  "Lateral"
  range -1800000000..  1800000001/1 -> Bus Creator1/6  "Longitudinal"
  SELF_Fiat_Bravo_1/1 -> SELF_Demux/1(SELF)
  J2735 Encoder Basic Safety Message/1(f()) -> DSRC Transmitter/Enable
  J2735 Encoder Basic Safety Message/2(Data) -> DSRC Transmitter/1(Data)
  DSRC Transmitter/1(DSRC_T) -> Memory/1
  Trajectories/1(State) -> STATE_Fiat_Bravo_1/1
  SELF_Demux/7(GPS lat [deg]) -> to micro degrees/1
  SELF_Demux/8(GPS long [deg]) -> to micro  degrees/1
  Bus Creator1/1 -> J2735 Encoder Basic Safety Message/1(Msg)
  SELF_Demux/1(x [m]) -> Terminator_1/1
  SELF_Demux/2(y [m]) -> Terminator_2/1
  SELF_Demux/3(z [m]) -> Terminator_3/1
  SELF_Demux/4(rotx [deg]) -> Terminator_4/1
  SELF_Demux/5(roty [deg]) -> Terminator_5/1
  SELF_Demux/6(rotz [deg]) -> Terminator_6/1
  SELF_Demux/9(GPS alt [m]) -> Terminator_7/1
  SELF_Demux/10(velocity [m/s]) -> Terminator_8/1
  SELF_Demux/11(heading [deg]) -> Terminator_9/1
  SELF_Demux/12(yaw rate [deg/s]) -> Terminator_10/1
  Pulse Generator/1 -> J2735 Encoder Basic Safety Message/Enable  "Submit clock"
  Memory/1 -> DSRC_Tx_1/1

== system Demo_DSRC_BSM_Message_cs/GetSensors ==
  dummy : Inport
  GetSensors : M-S-Function  FunctionName=GetSensorsBlock  Parameters=TimeStep NrOfSensors
  tag scope: SimCoreSensors=global
  wires:
  GetSensors/1 -> [SimCoreSensors]
  dummy/1 -> GetSensors/1

== system Demo_DSRC_BSM_Message_cs/SELF_BMW_Z3_1 ==
  Selector : Selector  IndexMode=Zero-based  IndexOptions=Starting index (dialog)  Indices=PortIndex  OutputSizes=PortWidth(1)
  U : Outport
  wires:
  Selector/1 -> U/1
  [SimCoreSensors] -> Selector/1

== system Demo_DSRC_BSM_Message_cs/SELF_Citroen_C3_1 ==
  Selector : Selector  IndexMode=Zero-based  IndexOptions=Starting index (dialog)  Indices=PortIndex  OutputSizes=PortWidth(1)
  U : Outport
  wires:
  Selector/1 -> U/1
  [SimCoreSensors] -> Selector/1

== system Demo_DSRC_BSM_Message_cs/SELF_Fiat_Bravo_1 ==
  Selector : Selector  IndexMode=Zero-based  IndexOptions=Starting index (dialog)  Indices=PortIndex  OutputSizes=PortWidth(1)
  U : Outport
  wires:
  Selector/1 -> U/1
  [SimCoreSensors] -> Selector/1

== system Demo_DSRC_BSM_Message_cs/STATE_BMW_Z3_1 ==
  State : Inport  SampleTime=TimeStep
  Acceleration : Subsystem  mask(ToSensorWorld){PortName=Acceleration_BMW_Z3_1, PortIndex=6, PortWidth=3, TimeStep=1/20}
      mask prompts: PortName "Port Name [-]"; PortIndex "Index [-]"; PortWidth "Port Dimensions [-]"; TimeStep "Upload Period [s]"
      mask help: Sends signal(s) from Simulink to the Sensor World
      mask Help:
      | Sends signal(s) from Simulink to the Sensor World.
      | 
      | - Port Name [-]: specifies the name of the output terminal of the Simulink block.
      | - Index [-]: specifies the start position in the output vector sent to the Sensor World
      | - Port dimensions [-]: specifies the width (number of scalars) of the output port
      | - Upload period [s]: specifies the upload period (in seconds) of the port.
      mask Display: port_label('input', 1, PortName)
  Demux : Demux  Outputs=5
  Position : Subsystem  mask(ToSensorWorld){PortName=Position_BMW_Z3_1, PortIndex=0, PortWidth=3, TimeStep=1/20}
      mask prompts: PortName "Port Name [-]"; PortIndex "Index [-]"; PortWidth "Port Dimensions [-]"; TimeStep "Upload Period [s]"
      mask help: Sends signal(s) from Simulink to the Sensor World
      mask Help:
      | Sends signal(s) from Simulink to the Sensor World.
      | 
      | - Port Name [-]: specifies the name of the output terminal of the Simulink block.
      | - Index [-]: specifies the start position in the output vector sent to the Sensor World
      | - Port dimensions [-]: specifies the width (number of scalars) of the output port
      | - Upload period [s]: specifies the upload period (in seconds) of the port.
      mask Display: port_label('input', 1, PortName)
  RPY : Subsystem  mask(ToSensorWorld){PortName=RPY_BMW_Z3_1, PortIndex=9, PortWidth=3, TimeStep=1/20}
      mask prompts: PortName "Port Name [-]"; PortIndex "Index [-]"; PortWidth "Port Dimensions [-]"; TimeStep "Upload Period [s]"
      mask help: Sends signal(s) from Simulink to the Sensor World
      mask Help:
      | Sends signal(s) from Simulink to the Sensor World.
      | 
      | - Port Name [-]: specifies the name of the output terminal of the Simulink block.
      | - Index [-]: specifies the start position in the output vector sent to the Sensor World
      | - Port dimensions [-]: specifies the width (number of scalars) of the output port
      | - Upload period [s]: specifies the upload period (in seconds) of the port.
      mask Display: port_label('input', 1, PortName)
  Velocity : Subsystem  mask(ToSensorWorld){PortName=Velocity_BMW_Z3_1, PortIndex=3, PortWidth=3, TimeStep=1/20}
      mask prompts: PortName "Port Name [-]"; PortIndex "Index [-]"; PortWidth "Port Dimensions [-]"; TimeStep "Upload Period [s]"
      mask help: Sends signal(s) from Simulink to the Sensor World
      mask Help:
      | Sends signal(s) from Simulink to the Sensor World.
      | 
      | - Port Name [-]: specifies the name of the output terminal of the Simulink block.
      | - Index [-]: specifies the start position in the output vector sent to the Sensor World
      | - Port dimensions [-]: specifies the width (number of scalars) of the output port
      | - Upload period [s]: specifies the upload period (in seconds) of the port.
      mask Display: port_label('input', 1, PortName)
  iniBODYAngles wrtVEH [rad] : Constant  Value=[Roll0 Pitch0 0]  SampleTime=TimeStep
  iniVEHAngles wrtGLOB [rad] : Constant  Value=[0 0 Yaw0]  SampleTime=TimeStep
  iniVEHposition wrtGLOB [m] : Constant  Value=[x0 y0 z0]  SampleTime=TimeStep
  state2FullState : PreScanSimulinkLibrary/state2FullState  SystemSampleTime=-1
  velRPY : Subsystem  mask(ToSensorWorld){PortName=velRPY_BMW_Z3_1, PortIndex=12, PortWidth=3, TimeStep=1/20}
      mask prompts: PortName "Port Name [-]"; PortIndex "Index [-]"; PortWidth "Port Dimensions [-]"; TimeStep "Upload Period [s]"
      mask help: Sends signal(s) from Simulink to the Sensor World
      mask Help:
      | Sends signal(s) from Simulink to the Sensor World.
      | 
      | - Port Name [-]: specifies the name of the output terminal of the Simulink block.
      | - Index [-]: specifies the start position in the output vector sent to the Sensor World
      | - Port dimensions [-]: specifies the width (number of scalars) of the output port
      | - Upload period [s]: specifies the upload period (in seconds) of the port.
      mask Display: port_label('input', 1, PortName)
  wires:
  Demux/5 -> velRPY/1(Y)
  Demux/4 -> RPY/1(Y)
  Demux/3 -> Acceleration/1(Y)
  Demux/2 -> Velocity/1(Y)
  Demux/1 -> Position/1(Y)
  State/1 -> state2FullState/1
  state2FullState/1 -> Demux/1
  iniVEHposition wrtGLOB [m]/1 -> state2FullState/2
  iniBODYAngles wrtVEH [rad]/1 -> state2FullState/3
  iniVEHAngles wrtGLOB [rad]/1 -> state2FullState/4

== system Demo_DSRC_BSM_Message_cs/STATE_Citroen_C3_1 ==
  State : Inport  SampleTime=TimeStep
  Acceleration : Subsystem  mask(ToSensorWorld){PortName=Acceleration_Citroen_C3_1, PortIndex=60, PortWidth=3, TimeStep=1/20}
      mask prompts: PortName "Port Name [-]"; PortIndex "Index [-]"; PortWidth "Port Dimensions [-]"; TimeStep "Upload Period [s]"
      mask help: Sends signal(s) from Simulink to the Sensor World
      mask Help:
      | Sends signal(s) from Simulink to the Sensor World.
      | 
      | - Port Name [-]: specifies the name of the output terminal of the Simulink block.
      | - Index [-]: specifies the start position in the output vector sent to the Sensor World
      | - Port dimensions [-]: specifies the width (number of scalars) of the output port
      | - Upload period [s]: specifies the upload period (in seconds) of the port.
      mask Display: port_label('input', 1, PortName)
  Demux : Demux  Outputs=5
  Position : Subsystem  mask(ToSensorWorld){PortName=Position_Citroen_C3_1, PortIndex=54, PortWidth=3, TimeStep=1/20}
      mask prompts: PortName "Port Name [-]"; PortIndex "Index [-]"; PortWidth "Port Dimensions [-]"; TimeStep "Upload Period [s]"
      mask help: Sends signal(s) from Simulink to the Sensor World
      mask Help:
      | Sends signal(s) from Simulink to the Sensor World.
      | 
      | - Port Name [-]: specifies the name of the output terminal of the Simulink block.
      | - Index [-]: specifies the start position in the output vector sent to the Sensor World
      | - Port dimensions [-]: specifies the width (number of scalars) of the output port
      | - Upload period [s]: specifies the upload period (in seconds) of the port.
      mask Display: port_label('input', 1, PortName)
  RPY : Subsystem  mask(ToSensorWorld){PortName=RPY_Citroen_C3_1, PortIndex=63, PortWidth=3, TimeStep=1/20}
      mask prompts: PortName "Port Name [-]"; PortIndex "Index [-]"; PortWidth "Port Dimensions [-]"; TimeStep "Upload Period [s]"
      mask help: Sends signal(s) from Simulink to the Sensor World
      mask Help:
      | Sends signal(s) from Simulink to the Sensor World.
      | 
      | - Port Name [-]: specifies the name of the output terminal of the Simulink block.
      | - Index [-]: specifies the start position in the output vector sent to the Sensor World
      | - Port dimensions [-]: specifies the width (number of scalars) of the output port
      | - Upload period [s]: specifies the upload period (in seconds) of the port.
      mask Display: port_label('input', 1, PortName)
  Velocity : Subsystem  mask(ToSensorWorld){PortName=Velocity_Citroen_C3_1, PortIndex=57, PortWidth=3, TimeStep=1/20}
      mask prompts: PortName "Port Name [-]"; PortIndex "Index [-]"; PortWidth "Port Dimensions [-]"; TimeStep "Upload Period [s]"
      mask help: Sends signal(s) from Simulink to the Sensor World
      mask Help:
      | Sends signal(s) from Simulink to the Sensor World.
      | 
      | - Port Name [-]: specifies the name of the output terminal of the Simulink block.
      | - Index [-]: specifies the start position in the output vector sent to the Sensor World
      | - Port dimensions [-]: specifies the width (number of scalars) of the output port
      | - Upload period [s]: specifies the upload period (in seconds) of the port.
      mask Display: port_label('input', 1, PortName)
  iniBODYAngles wrtVEH [rad] : Constant  Value=[Roll0 Pitch0 0]  SampleTime=TimeStep
  iniVEHAngles wrtGLOB [rad] : Constant  Value=[0 0 Yaw0]  SampleTime=TimeStep
  iniVEHposition wrtGLOB [m] : Constant  Value=[x0 y0 z0]  SampleTime=TimeStep
  state2FullState : PreScanSimulinkLibrary/state2FullState  SystemSampleTime=-1
  velRPY : Subsystem  mask(ToSensorWorld){PortName=velRPY_Citroen_C3_1, PortIndex=66, PortWidth=3, TimeStep=1/20}
      mask prompts: PortName "Port Name [-]"; PortIndex "Index [-]"; PortWidth "Port Dimensions [-]"; TimeStep "Upload Period [s]"
      mask help: Sends signal(s) from Simulink to the Sensor World
      mask Help:
      | Sends signal(s) from Simulink to the Sensor World.
      | 
      | - Port Name [-]: specifies the name of the output terminal of the Simulink block.
      | - Index [-]: specifies the start position in the output vector sent to the Sensor World
      | - Port dimensions [-]: specifies the width (number of scalars) of the output port
      | - Upload period [s]: specifies the upload period (in seconds) of the port.
      mask Display: port_label('input', 1, PortName)
  wires:
  Demux/5 -> velRPY/1(Y)
  Demux/4 -> RPY/1(Y)
  Demux/3 -> Acceleration/1(Y)
  Demux/2 -> Velocity/1(Y)
  Demux/1 -> Position/1(Y)
  State/1 -> state2FullState/1
  state2FullState/1 -> Demux/1
  iniVEHposition wrtGLOB [m]/1 -> state2FullState/2
  iniBODYAngles wrtVEH [rad]/1 -> state2FullState/3
  iniVEHAngles wrtGLOB [rad]/1 -> state2FullState/4

== system Demo_DSRC_BSM_Message_cs/STATE_Fiat_Bravo_1 ==
  State : Inport  SampleTime=TimeStep
  Acceleration : Subsystem  mask(ToSensorWorld){PortName=Acceleration_Fiat_Bravo_1, PortIndex=21, PortWidth=3, TimeStep=1/20}
      mask prompts: PortName "Port Name [-]"; PortIndex "Index [-]"; PortWidth "Port Dimensions [-]"; TimeStep "Upload Period [s]"
      mask help: Sends signal(s) from Simulink to the Sensor World
      mask Help:
      | Sends signal(s) from Simulink to the Sensor World.
      | 
      | - Port Name [-]: specifies the name of the output terminal of the Simulink block.
      | - Index [-]: specifies the start position in the output vector sent to the Sensor World
      | - Port dimensions [-]: specifies the width (number of scalars) of the output port
      | - Upload period [s]: specifies the upload period (in seconds) of the port.
      mask Display: port_label('input', 1, PortName)
  Demux : Demux  Outputs=5
  Position : Subsystem  mask(ToSensorWorld){PortName=Position_Fiat_Bravo_1, PortIndex=15, PortWidth=3, TimeStep=1/20}
      mask prompts: PortName "Port Name [-]"; PortIndex "Index [-]"; PortWidth "Port Dimensions [-]"; TimeStep "Upload Period [s]"
      mask help: Sends signal(s) from Simulink to the Sensor World
      mask Help:
      | Sends signal(s) from Simulink to the Sensor World.
      | 
      | - Port Name [-]: specifies the name of the output terminal of the Simulink block.
      | - Index [-]: specifies the start position in the output vector sent to the Sensor World
      | - Port dimensions [-]: specifies the width (number of scalars) of the output port
      | - Upload period [s]: specifies the upload period (in seconds) of the port.
      mask Display: port_label('input', 1, PortName)
  RPY : Subsystem  mask(ToSensorWorld){PortName=RPY_Fiat_Bravo_1, PortIndex=24, PortWidth=3, TimeStep=1/20}
      mask prompts: PortName "Port Name [-]"; PortIndex "Index [-]"; PortWidth "Port Dimensions [-]"; TimeStep "Upload Period [s]"
      mask help: Sends signal(s) from Simulink to the Sensor World
      mask Help:
      | Sends signal(s) from Simulink to the Sensor World.
      | 
      | - Port Name [-]: specifies the name of the output terminal of the Simulink block.
      | - Index [-]: specifies the start position in the output vector sent to the Sensor World
      | - Port dimensions [-]: specifies the width (number of scalars) of the output port
      | - Upload period [s]: specifies the upload period (in seconds) of the port.
      mask Display: port_label('input', 1, PortName)
  Velocity : Subsystem  mask(ToSensorWorld){PortName=Velocity_Fiat_Bravo_1, PortIndex=18, PortWidth=3, TimeStep=1/20}
      mask prompts: PortName "Port Name [-]"; PortIndex "Index [-]"; PortWidth "Port Dimensions [-]"; TimeStep "Upload Period [s]"
      mask help: Sends signal(s) from Simulink to the Sensor World
      mask Help:
      | Sends signal(s) from Simulink to the Sensor World.
      | 
      | - Port Name [-]: specifies the name of the output terminal of the Simulink block.
      | - Index [-]: specifies the start position in the output vector sent to the Sensor World
      | - Port dimensions [-]: specifies the width (number of scalars) of the output port
      | - Upload period [s]: specifies the upload period (in seconds) of the port.
      mask Display: port_label('input', 1, PortName)
  iniBODYAngles wrtVEH [rad] : Constant  Value=[Roll0 Pitch0 0]  SampleTime=TimeStep
  iniVEHAngles wrtGLOB [rad] : Constant  Value=[0 0 Yaw0]  SampleTime=TimeStep
  iniVEHposition wrtGLOB [m] : Constant  Value=[x0 y0 z0]  SampleTime=TimeStep
  state2FullState : PreScanSimulinkLibrary/state2FullState  SystemSampleTime=-1
  velRPY : Subsystem  mask(ToSensorWorld){PortName=velRPY_Fiat_Bravo_1, PortIndex=27, PortWidth=3, TimeStep=1/20}
      mask prompts: PortName "Port Name [-]"; PortIndex "Index [-]"; PortWidth "Port Dimensions [-]"; TimeStep "Upload Period [s]"
      mask help: Sends signal(s) from Simulink to the Sensor World
      mask Help:
      | Sends signal(s) from Simulink to the Sensor World.
      | 
      | - Port Name [-]: specifies the name of the output terminal of the Simulink block.
      | - Index [-]: specifies the start position in the output vector sent to the Sensor World
      | - Port dimensions [-]: specifies the width (number of scalars) of the output port
      | - Upload period [s]: specifies the upload period (in seconds) of the port.
      mask Display: port_label('input', 1, PortName)
  wires:
  Demux/5 -> velRPY/1(Y)
  Demux/4 -> RPY/1(Y)
  Demux/3 -> Acceleration/1(Y)
  Demux/2 -> Velocity/1(Y)
  Demux/1 -> Position/1(Y)
  State/1 -> state2FullState/1
  state2FullState/1 -> Demux/1
  iniVEHposition wrtGLOB [m]/1 -> state2FullState/2
  iniBODYAngles wrtVEH [rad]/1 -> state2FullState/3
  iniVEHAngles wrtGLOB [rad]/1 -> state2FullState/4

== system Demo_DSRC_BSM_Message_cs/SetActuators ==
  Bus Creator : BusCreator  Inputs=1
  Data Store Read : DataStoreRead  DataStoreName=SimCoreActuators  SampleTime=TimeStep
  SendActuators : M-S-Function  FunctionName=SendActuatorsBlock  Parameters=TimeStep NrOfActuators
  dummy : Outport
  tag scope: SimCoreInfo=global
  wires:
  Bus Creator/1 -> [SimCoreInfo]  "SimCore"
  SendActuators/2 -> Bus Creator/1  "ComputationTime[s]"
  SendActuators/1 -> dummy/1
  Data Store Read/1 -> SendActuators/1

== system Demo_DSRC_BSM_Message_cs/SimCoreInfo ==
  Bus Selector : BusSelector  OutputSignals=ComputationTime[s]
  Time : Scope
      settings: TimeRange=10  YMin=0  YMax=0.5  SaveName=ComputationTime
  wires:
  Bus Selector/1 -> Time/1  "<ComputationTime[s]>"
  [SimCoreInfo] -> Bus Selector/1

== system Demo_DSRC_BSM_Message_cs/BMW_Z3_1/DSRC Receiver ==
  In1 : Inport
  Always Enabled : Constant
  Bus Selector : BusSelector  OutputSignals=spare_1,spare_2,spare_3,spare_4,spare_5,spare_6,spare_7,spare_8,spare_9,spare_10,spare_11,spare_12,spare_13,spare_14,spare_15,spare_16,spare_17,spare_18,spare_19  OutputAsBus=on
  Bus to Vector : BusToVector
  DSRC_Rx_Demux : Subsystem  Tag=DemuxDSRCR
      settings: DeleteFcn=PreScanBlockDeleteFcn;
      mask Type: PreScan Demux Block:
      mask Display:
      | port_label('output', 1, 'Vehicle_ID')
      | port_label('output', 2, 'GPS Pos Lat [deg]')
      | port_label('output', 3, 'GPS Pos Long [deg]')
      | port_label('output', 4, 'GPS Pos Alt [m]')
      | port_label('output', 5, 'Velocity [m/s]')
      | port_label('output', 6, 'Acceleration [m/s2]')
      | port_label('output', 7, 'Heading [deg]')
      | port_label('output', 8, 'Warning signal ID')
      | port_label('output', 9, 'Maneuvre ID')
      | port_label('output', 10, 'Vehicle Type')
      | port_label('output', 11, 'Braking Capacity')
      | port_label('output', 12, 'Vehicle Size')
      | port_label('output', 13, 'Spare')
  Terminator_{2..13} (12 alike) : Terminator
  f() : Outport
  Data : Outport  Port=2
  wires:
  Bus to Vector/1 -> Data/1
  Bus Selector/1 -> Bus to Vector/1
  DSRC_Rx_Demux/13(spare) -> Bus Selector/1  "L7"
  Always Enabled/1 -> f()/1  "Enable"
  In1/1 -> DSRC_Rx_Demux/1(AntennaR)
  DSRC_Rx_Demux/12(vehicle_size) -> Terminator_13/1
  DSRC_Rx_Demux/11(brakingcapacity) -> Terminator_12/1
  DSRC_Rx_Demux/10(vehicle_type) -> Terminator_11/1
  DSRC_Rx_Demux/9(maneuvre_id) -> Terminator_10/1
  DSRC_Rx_Demux/8(warning_signal_id) -> Terminator_9/1
  DSRC_Rx_Demux/7(Heading [deg]) -> Terminator_8/1
  DSRC_Rx_Demux/6(Acceleration_[m/s2]) -> Terminator_7/1
  DSRC_Rx_Demux/5(Velocity_[m/s]) -> Terminator_6/1
  DSRC_Rx_Demux/4(GPS_pos_alt_[m]) -> Terminator_5/1
  DSRC_Rx_Demux/3(GPS_pos_long_[deg]) -> Terminator_4/1
  DSRC_Rx_Demux/2(GPS_pos_lat_[deg]) -> Terminator_3/1
  DSRC_Rx_Demux/1(Vehicle_ID) -> Terminator_2/1

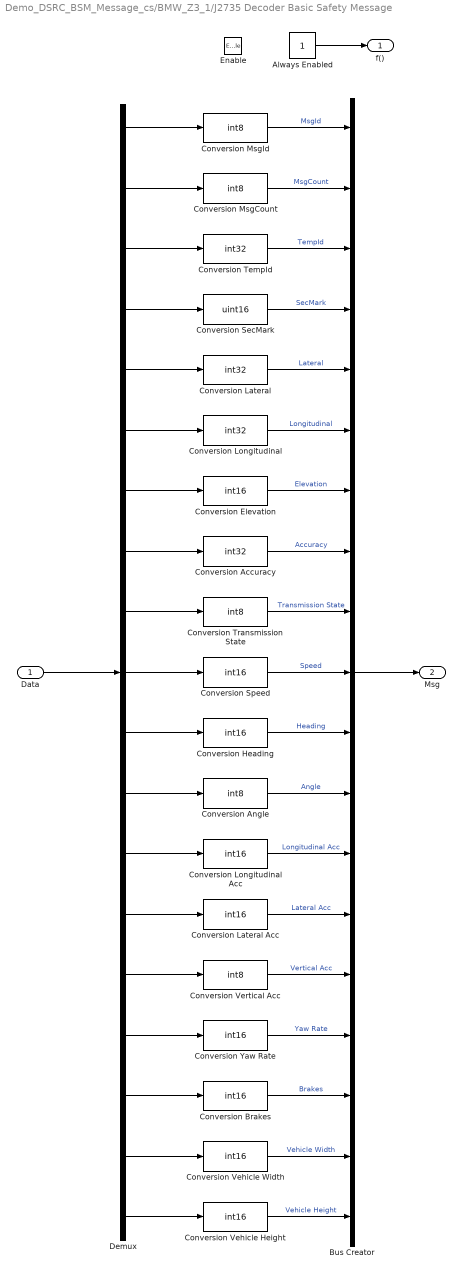
== system Demo_DSRC_BSM_Message_cs/BMW_Z3_1/J2735 Decoder Basic Safety Message ==
  Data : Inport
  Enable : EnablePort  PropagateVarSize=During execution
  Always Enabled : Constant
  Bus Creator : BusCreator  Inputs=19
  Conversion Accuracy : DataTypeConversion  OutDataTypeStr=int32
  Conversion Angle : DataTypeConversion  OutDataTypeStr=int8
  Conversion Brakes : DataTypeConversion  OutDataTypeStr=int16
  Conversion Elevation : DataTypeConversion  OutDataTypeStr=int16
  Conversion Heading : DataTypeConversion  OutDataTypeStr=int16
  Conversion Lateral : DataTypeConversion  OutDataTypeStr=int32
  Conversion Lateral Acc : DataTypeConversion  OutDataTypeStr=int16
  Conversion Longitudinal : DataTypeConversion  OutDataTypeStr=int32
  Conversion Longitudinal Acc : DataTypeConversion  OutDataTypeStr=int16
  Conversion MsgCount : DataTypeConversion  OutDataTypeStr=int8
  Conversion MsgId : DataTypeConversion  OutDataTypeStr=int8
  Conversion SecMark : DataTypeConversion  OutDataTypeStr=uint16
  Conversion Speed : DataTypeConversion  OutDataTypeStr=int16
  Conversion TempId : DataTypeConversion  OutDataTypeStr=int32
  Conversion Transmission State : DataTypeConversion  OutDataTypeStr=int8
  Conversion Vehicle Height : DataTypeConversion  OutDataTypeStr=int16
  Conversion Vehicle Width : DataTypeConversion  OutDataTypeStr=int16
  Conversion Vertical Acc : DataTypeConversion  OutDataTypeStr=int8
  Conversion Yaw Rate : DataTypeConversion  OutDataTypeStr=int16
  Demux : Demux  Outputs=19
  f() : Outport  InitialOutput=[1]
  Msg : Outport  Port=2
  wires:
  Conversion Vehicle Height/1 -> Bus Creator/19  "Vehicle Height"
  Demux/19 -> Conversion Vehicle Height/1
  Conversion Vehicle Width/1 -> Bus Creator/18  "Vehicle Width"
  Conversion Brakes/1 -> Bus Creator/17  "Brakes"
  Demux/18 -> Conversion Vehicle Width/1
  Demux/17 -> Conversion Brakes/1
  Conversion Yaw Rate/1 -> Bus Creator/16  "Yaw Rate"
  Conversion Vertical Acc/1 -> Bus Creator/15  "Vertical Acc"
  Demux/16 -> Conversion Yaw Rate/1
  Demux/15 -> Conversion Vertical Acc/1
  Conversion Lateral Acc/1 -> Bus Creator/14  "Lateral Acc"
  Conversion Longitudinal Acc/1 -> Bus Creator/13  "Longitudinal Acc"
  Demux/14 -> Conversion Lateral Acc/1
  Demux/13 -> Conversion Longitudinal Acc/1
  Conversion Angle/1 -> Bus Creator/12  "Angle"
  Conversion Heading/1 -> Bus Creator/11  "Heading"
  Demux/12 -> Conversion Angle/1
  Demux/11 -> Conversion Heading/1
  Conversion Speed/1 -> Bus Creator/10  "Speed"
  Conversion Transmission State/1 -> Bus Creator/9  "Transmission State"
  Demux/10 -> Conversion Speed/1
  Demux/9 -> Conversion Transmission State/1
  Conversion Accuracy/1 -> Bus Creator/8  "Accuracy"
  Demux/8 -> Conversion Accuracy/1
  Conversion Elevation/1 -> Bus Creator/7  "Elevation"
  Demux/7 -> Conversion Elevation/1
  Conversion Longitudinal/1 -> Bus Creator/6  "Longitudinal"
  Demux/6 -> Conversion Longitudinal/1
  Conversion Lateral/1 -> Bus Creator/5  "Lateral"
  Demux/5 -> Conversion Lateral/1
  Conversion SecMark/1 -> Bus Creator/4  "SecMark"
  Demux/4 -> Conversion SecMark/1
  Conversion TempId/1 -> Bus Creator/3  "TempId"
  Demux/3 -> Conversion TempId/1
  Demux/2 -> Conversion MsgCount/1
  Conversion MsgCount/1 -> Bus Creator/2  "MsgCount"
  Bus Creator/1 -> Msg/1
  Conversion MsgId/1 -> Bus Creator/1  "MsgId"
  Demux/1 -> Conversion MsgId/1
  Data/1 -> Demux/1
  Always Enabled/1 -> f()/1
